simulink model "SD2231_Lab1_2022"  (R2020b)
settings: Solver=VariableStepAuto  StartTime=0.0  StopTime=inf  RelTol=1e-3
values from neighbouring files (symbols this model uses):
  K_awup = Ki_br_r/Kp_br_r    (= 10.4166666667)    [initial.m]
  K_brake = K_brake(3)    [initial.m]
  K_em = K_em(3)    [initial.m]
  Kd_br_f = 0.6*T_new_rl_b    (= 0.1722)    [initial.m]
  Kd_br_r = 0.6*T_new_rl_b    (= 0.1722)    [initial.m]
  Kd_tr = 0.6*T_new    (= 0.0093)    [initial.m]
  Ki_br_f = 0.6*T_new_rl_b/L_new_rl_b^2    (= 74.7395833333)    [initial.m]
  Ki_br_r = 0.6*T_new_rl_b/L_new_rl_b^2    (= 74.7395833333)    [initial.m]
  Ki_tr = 2*T_new/L_new^2    (= 13.7396121884)    [initial.m]
  Kp_br_f = 2*1.2*T_new_rl_b/L_new_rl_b    (= 14.35)    [initial.m]
  Kp_br_r = 1.2*T_new_rl_b/L_new_rl_b    (= 7.175)    [initial.m]
  Kp_tr = 4*1.2*T_new/L_new    (= 1.56631578947)    [initial.m]
  low_th_zeroDiv = 0.5    [initial.m]
  N = 100    [initial.m]
  ref_br_f = 0.15    [initial.m]
  ref_br_r = 0.17    [initial.m]
  ref_tr = 0.06    [initial.m]
  step_time = 2    [initial.m]
  threshold_br_f = ref_br_f-0.05    (= 0.1)    [initial.m]
  threshold_br_r = ref_br_r-0.05    (= 0.12)    [initial.m]
  threshold_tc = ref_tr-0.02    (= 0.04)    [initial.m]
  vx_threshold = 1    [initial.m]
undefined symbols (not defined in the file or in its folder): DiscIntNeverNeededParam, Veh
libraries: CarMaker4SL x38, simulink x2, autolibmappedmotor x2
(part 4 of 4)

== matlab function SD2231_Lab1_2022/CarMaker/Your ABS Controller/Activation Logic Br RR/controller/PID1/MATLAB Function ==
  data: threshold_br_r input; slip input; Brk input; res output
function res = fcn(threshold_br_r, slip, Brk)
if Brk >0 && slip > threshold_br_r
    res = 1;
else
    res = 0;
end
end

== matlab function SD2231_Lab1_2022/CarMaker/Your ABS Controller/Activation Logic Br FR/controller/PID1/MATLAB Function1 ==
  data: threshold_br_r input; slip input; Brk input; res output
function res = fcn(threshold_br_r, slip, Brk)
if Brk >0 && slip > threshold_br_r
    res = 1;
else
    res = 0;
end
end

== matlab function SD2231_Lab1_2022/CarMaker/Road friction/MATLAB Function ==
  data: vx input; mu output; ax input
function mu = fcn(vx, ax)
    if vx > 10 && ax > 0 && vx<20
        mu = 0.7;
    elseif vx < 10 && ax <-0.3 
        mu = 0.3;
    else
        mu = 1;
    end

== matlab function SD2231_Lab1_2022/CarMaker/Your Traction Controller/Activation Logic Tr RL/MATLAB Function ==
  settings: updateMethod=DISCRETE
  data: ax input; Thr input; slip input; AdjThr input; y output; threshold input; dbg output
function [y,dbg] = fcn(ax, Thr,slip,AdjThr,threshold)

if Thr > 0 && ax >0 && slip > threshold 
    if AdjThr > 0
        AdjThr = 0;
    end
    y = AdjThr+Thr;
    dbg = 1;   
else
    
    y = Thr;
    %For later, try without this line
    dbg = 0;
end

== matlab function SD2231_Lab1_2022/CarMaker/Your Traction Controller/Activation Logic Tr RL/controller/PID1/MATLAB Function ==
  data: threshold input; slip input; Thr input; res output
function res = fcn(threshold, slip, Thr)
if Thr >0 && slip > threshold
    res = 1;
else
    res = 0;
end
end

== matlab function SD2231_Lab1_2022/CarMaker/Your Traction Controller/Activation Logic Tr RR/controller/PID1/MATLAB Function ==
  data: threshold input; slip input; Thr input; res output
function res = fcn(threshold, slip, Thr)
if Thr >0 && slip > threshold
    res = 1;
else
    res = 0;
end
end

== matlab function SD2231_Lab1_2022/CarMaker/Your Traction Controller/Activation Logic Tr RR/MATLAB Function ==
  data: ax input; Thr input; slip input; AdjThr input; y output; threshold input
    function y = fcn(ax, Thr,slip,AdjThr, threshold)
if Thr > 0 && ax >0 && slip > threshold 
    if AdjThr >0
        AdjThr = 0;
    end
    
    y = AdjThr+Thr;
else 
    y = Thr; %For later, try without this line
end

== matlab function SD2231_Lab1_2022/CarMaker/Your ABS Controller/Activation Logic Br FL/MATLAB Function ==
  data: vx input; ax input; Brk input; slip input; AdjBrk input; y output; threshold input; vx_threshold input
function y = fcn(vx, ax, Brk,slip,AdjBrk, threshold,vx_threshold)
if Brk > 0 && ax <0 && slip > threshold && vx > vx_threshold
    if AdjBrk > 0
        AdjBrk = 0;
    end
    y = AdjBrk+Brk;
else 
    y = Brk; %For later, try without this line
end

== matlab function SD2231_Lab1_2022/CarMaker/Your ABS Controller/Activation Logic Br FL/controller/PID1/MATLAB Function ==
  data: threshold_br_r input; slip input; Brk input; res output
function res = fcn(threshold_br_r, slip, Brk)
if Brk >0 && slip > threshold_br_r
    res = 1;
else
    res = 0;
end
end

== matlab function SD2231_Lab1_2022/CarMaker/Your ABS Controller/Activation Logic Br FR/MATLAB Function ==
  data: vx input; ax input; Brk input; slip input; AdjBrk input; y output; threshold input; vx_threshold input
function y = fcn(vx, ax, Brk,slip,AdjBrk, threshold,vx_threshold)
if Brk > 0 && ax <0 && slip > threshold && vx > vx_threshold
    if AdjBrk > 0
        AdjBrk = 0;
    end
    y = AdjBrk+Brk;
else 
    y = Brk; %For later, try without this line
end

== matlab function SD2231_Lab1_2022/CarMaker/Your Traction Controller/Activation Logic Tr RR/controller/PID/MATLAB Function1 ==
  data: Thr input; res output; threshold input; slip input
function res = fcn(Thr,threshold,slip)
if Thr >0 && slip > threshold
    res = 1;
else
    res = 0;
end
end

== matlab function SD2231_Lab1_2022/CarMaker/Your ABS Controller/Activation Logic Br RL/MATLAB Function ==
  data: vx input; ax input; Brk input; slip input; AdjBrk input; y output; threshold input; vx_threshold input
function y = fcn(vx, ax, Brk,slip,AdjBrk, threshold,vx_threshold)
if Brk > 0 && ax <0 && slip > threshold && vx > vx_threshold
    if AdjBrk > 0
        AdjBrk = 0;
    end
    y = AdjBrk+Brk;
else 
    y = Brk; %For later, try without this line
end

== matlab function SD2231_Lab1_2022/CarMaker/Your ABS Controller/Activation Logic Br RL/controller/PID1/MATLAB Function ==
  data: threshold_br_r input; slip input; Brk input; res output
function res = fcn(threshold_br_r, slip, Brk)
if Brk >0 && slip > threshold_br_r
    res = 1;
else
    res = 0;
end
end
